simulink model "CompleteModel"  (R2015b)
settings: Solver=VariableStepAuto  StartTime=0.0  StopTime=t  RelTol=1e-3
undefined symbols (not defined in the file): Fg, Jx, Jy, Jz, kd, kth, L, m, w1_bar, w2_bar, w3_bar, w4_bar
libraries: simulink x6
settings Model: Creator=USUARIO  LastModifiedBy=USUARIO

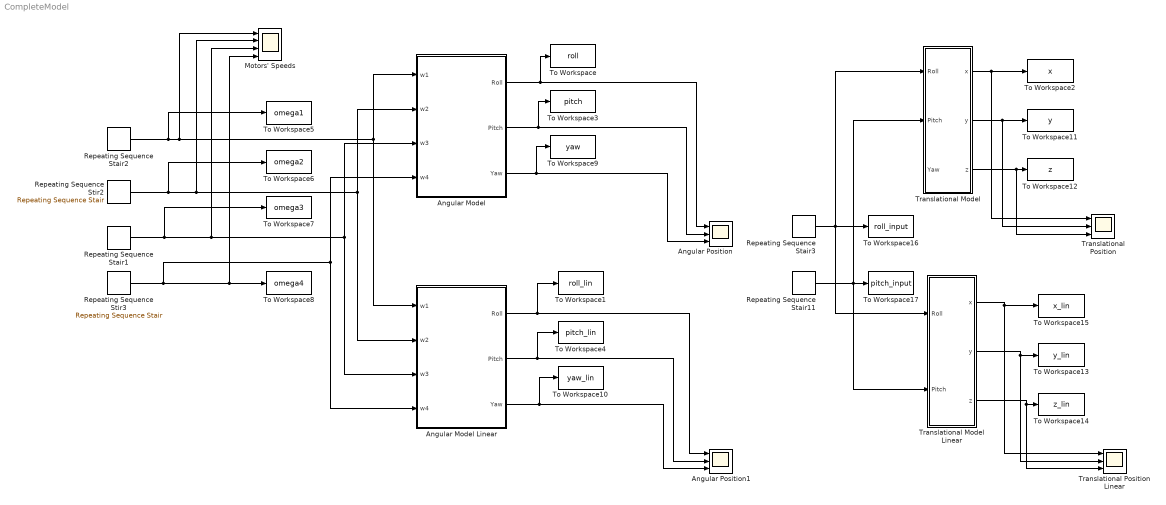
== system CompleteModel ==
  Angular Model : Subsystem
  Angular Model Linear : Subsystem
  Angular Position : Scope  NumInputPorts=3
  Angular Position1 : Scope  NumInputPorts=3
  Motors' Speeds : Scope  NumInputPorts=4
  Repeating Sequence Stair1 : simulink/Sources/Repeating Sequence Stair  OutValues=inputw3  tsamp=2  OutMin=[]  OutMax=[]  OutDataTypeStr=double  OutputDataTypeScalingMode=double  OutDataType=fixdt(0,8)  ConRadixGroup=Best Precision: Vector-wise  OutScaling=2^-12
  "Repeating Sequence Stair11 " : simulink/Sources/Repeating Sequence Stair  OutValues=inputpitch  tsamp=2  OutMin=[]  OutMax=[]  OutDataTypeStr=double  OutputDataTypeScalingMode=double  OutDataType=fixdt(0,8)  ConRadixGroup=Best Precision: Vector-wise  OutScaling=2^-12
  Repeating Sequence Stair2 : simulink/Sources/Repeating Sequence Stair  OutValues=inputw1  tsamp=2  OutMin=[]  OutMax=[]  OutDataTypeStr=double  OutputDataTypeScalingMode=double  OutDataType=fixdt(0,8)  ConRadixGroup=Best Precision: Vector-wise  OutScaling=2^-12
  Repeating Sequence Stair3 : simulink/Sources/Repeating Sequence Stair  OutValues=inputroll  tsamp=2  OutMin=[]  OutMax=[]  OutDataTypeStr=double  OutputDataTypeScalingMode=double  OutDataType=fixdt(0,8)  ConRadixGroup=Best Precision: Vector-wise  OutScaling=2^-12
  Repeating Sequence Stir2 : simulink/Sources/Repeating Sequence Stair  OutValues=inputw2  tsamp=2  OutMin=[]  OutMax=[]  OutDataTypeStr=double  OutputDataTypeScalingMode=double  OutDataType=fixdt(0,8)  ConRadixGroup=Best Precision: Vector-wise  OutScaling=2^-12
  Repeating Sequence Stir3 : simulink/Sources/Repeating Sequence Stair  OutValues=inputw4  tsamp=2  OutMin=[]  OutMax=[]  OutDataTypeStr=double  OutputDataTypeScalingMode=double  OutDataType=fixdt(0,8)  ConRadixGroup=Best Precision: Vector-wise  OutScaling=2^-12
  To Workspace : ToWorkspace  VariableName=roll  SaveFormat=Timeseries  SampleTime=0.1
  To Workspace1 : ToWorkspace  VariableName=roll_lin  SaveFormat=Timeseries  SampleTime=0.1
  To Workspace10 : ToWorkspace  VariableName=yaw_lin  SaveFormat=Timeseries  SampleTime=0.1
  To Workspace11 : ToWorkspace  VariableName=y  SaveFormat=Timeseries  SampleTime=0.1
  To Workspace12 : ToWorkspace  VariableName=z  SaveFormat=Timeseries  SampleTime=0.1
  To Workspace13 : ToWorkspace  VariableName=y_lin  SaveFormat=Timeseries  SampleTime=0.1
  To Workspace14 : ToWorkspace  VariableName=z_lin  SaveFormat=Timeseries  SampleTime=0.1
  To Workspace15 : ToWorkspace  VariableName=x_lin  SaveFormat=Timeseries  SampleTime=0.1
  To Workspace16 : ToWorkspace  VariableName=roll_input  SaveFormat=Timeseries  SampleTime=0.1
  To Workspace17 : ToWorkspace  VariableName=pitch_input  SaveFormat=Timeseries  SampleTime=0.1
  To Workspace2 : ToWorkspace  VariableName=x  SaveFormat=Timeseries  SampleTime=0.1
  To Workspace3 : ToWorkspace  VariableName=pitch  SaveFormat=Timeseries  SampleTime=0.1
  To Workspace4 : ToWorkspace  VariableName=pitch_lin  SaveFormat=Timeseries  SampleTime=0.1
  To Workspace5 : ToWorkspace  VariableName=omega1  SaveFormat=Timeseries  SampleTime=0.1
  To Workspace6 : ToWorkspace  VariableName=omega2  SaveFormat=Timeseries  SampleTime=0.1
  To Workspace7 : ToWorkspace  VariableName=omega3  SaveFormat=Timeseries  SampleTime=0.1
  To Workspace8 : ToWorkspace  VariableName=omega4  SaveFormat=Timeseries  SampleTime=0.1
  To Workspace9 : ToWorkspace  VariableName=yaw  SaveFormat=Timeseries  SampleTime=0.1
  Translational Model : Subsystem
  Translational Model Linear : Subsystem
  Translational Position : Scope  NumInputPorts=3
  Translational Position Linear : Scope  NumInputPorts=3
  wires:
  Angular Model/1(Roll) -> Angular Position/1, To Workspace/1
  Angular Model/2(Pitch) -> Angular Position/2, To Workspace3/1
  Angular Model/3(Yaw) -> To Workspace9/1, Angular Position/3
  Translational Model/1(x) -> To Workspace2/1, Translational Position/1
  Translational Model/2(y) -> To Workspace11/1, Translational Position/2
  Translational Model/3(z) -> Translational Position/3, To Workspace12/1
  Angular Model Linear/1(Roll) -> Angular Position1/1, To Workspace1/1
  Angular Model Linear/2(Pitch) -> To Workspace4/1, Angular Position1/2
  Angular Model Linear/3(Yaw) -> Angular Position1/3, To Workspace10/1
  Repeating Sequence Stir3/1 -> Motors' Speeds/4, To Workspace8/1, Angular Model/4(w4), Angular Model Linear/4(w4)
  Repeating Sequence Stair1/1 -> To Workspace7/1, Motors' Speeds/3, Angular Model/3(w3), Angular Model Linear/3(w3)
  Repeating Sequence Stir2/1 -> To Workspace6/1, Motors' Speeds/2, Angular Model Linear/2(w2), Angular Model/2(w2)
  Repeating Sequence Stair2/1 -> To Workspace5/1, Motors' Speeds/1, Angular Model Linear/1(w1), Angular Model/1(w1)
  Repeating Sequence Stair3/1 -> To Workspace16/1, Translational Model/1(Roll), Translational Model Linear/1(Roll)
  "Repeating Sequence Stair11 "/1 -> Translational Model/2(Pitch), To Workspace17/1, Translational Model Linear/2(Pitch)
  Translational Model Linear/1(x) -> Translational Position Linear/1, To Workspace15/1
  Translational Model Linear/2(y) -> Translational Position Linear/2, To Workspace13/1
  Translational Model Linear/3(z) -> Translational Position Linear/3, To Workspace14/1

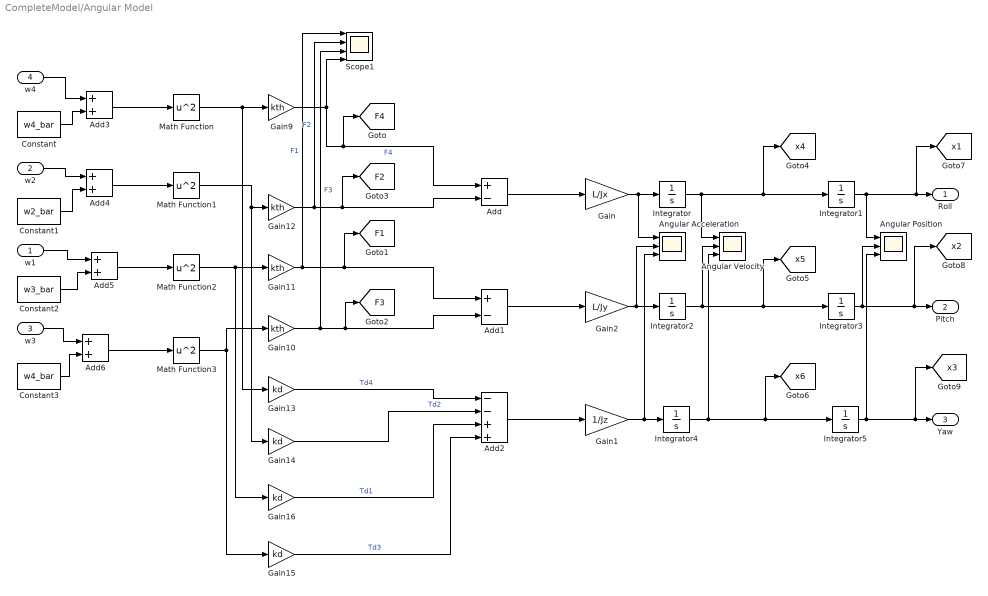
== system CompleteModel/Angular Model ==
  w1 : Inport
  w2 : Inport  Port=2
  w3 : Inport  Port=3
  w4 : Inport  Port=4
  Add : Sum  Inputs=+-
  Add1 : Sum  Inputs=+-
  Add2 : Sum  Inputs=--++
  Add{3..6} (4 alike) : Sum
  Angular Position : Scope  NumInputPorts=3
  Angular Velocity : Scope  NumInputPorts=3
  Angular Acceleration : Scope  NumInputPorts=3
  Constant : Constant  Value=w4_bar
  Constant1 : Constant  Value=w2_bar
  Constant2 : Constant  Value=w3_bar
  Constant3 : Constant  Value=w4_bar
  Gain : Gain  Gain=L/Jx
  Gain1 : Gain  Gain=1/Jz
  Gain{9..12} (4 alike) : Gain  Gain=kth
  Gain{13..16} (4 alike) : Gain  Gain=kd
  Gain2 : Gain  Gain=L/Jy
  Integrator{,1..5} (6 alike) : Integrator
  Math Function{,1..3} (4 alike) : Math  Operator=square  SaturateOnIntegerOverflow=on
  Scope1 : Scope  NumInputPorts=4
  Roll : Outport
  Pitch : Outport  Port=2
  Yaw : Outport  Port=3
  tag scope: F1=global, F2=global, F3=global, F4=global, x1=global, x2=global, x3=global, x4=global, x5=global, x6=global
  wires:
  Gain2/1 -> Angular Acceleration/2, Integrator2/1
  Add2/1 -> Gain1/1
  Gain9/1 -> [F4], Add/1, Scope1/4  "F4"
  Gain14/1 -> Add2/2  "Td2"
  Gain16/1 -> Add2/3  "Td1"
  Gain/1 -> Angular Acceleration/1, Integrator/1
  Integrator/1 -> Angular Velocity/1, Integrator1/1, [x4]
  Integrator1/1 -> [x1], Roll/1, Angular Position/1
  Integrator4/1 -> Angular Velocity/3, [x6], Integrator5/1
  Add/1 -> Gain/1
  Integrator3/1 -> [x2], Pitch/1, Angular Position/2
  Add1/1 -> Gain2/1
  Integrator5/1 -> Angular Position/3, [x3], Yaw/1
  Gain12/1 -> Scope1/2, [F2], Add/2  "F2"
  Gain10/1 -> [F3], Add1/2, Scope1/3  "F3"
  Gain11/1 -> Scope1/1, [F1], Add1/1  "F1"
  Gain13/1 -> Add2/1  "Td4"
  Gain15/1 -> Add2/4  "Td3"
  Integrator2/1 -> Angular Velocity/2, [x5], Integrator3/1
  Gain1/1 -> Angular Acceleration/3, Integrator4/1
  Math Function3/1 -> Gain10/1, Gain15/1
  Math Function2/1 -> Gain16/1, Gain11/1
  Math Function/1 -> Gain13/1, Gain9/1
  Math Function1/1 -> Gain14/1, Gain12/1
  w4/1 -> Add3/1
  Add3/1 -> Math Function/1
  Constant/1 -> Add3/2
  w2/1 -> Add4/1
  Add4/1 -> Math Function1/1
  Constant1/1 -> Add4/2
  w1/1 -> Add5/1
  Add5/1 -> Math Function2/1
  Constant2/1 -> Add5/2
  w3/1 -> Add6/1
  Add6/1 -> Math Function3/1
  Constant3/1 -> Add6/2

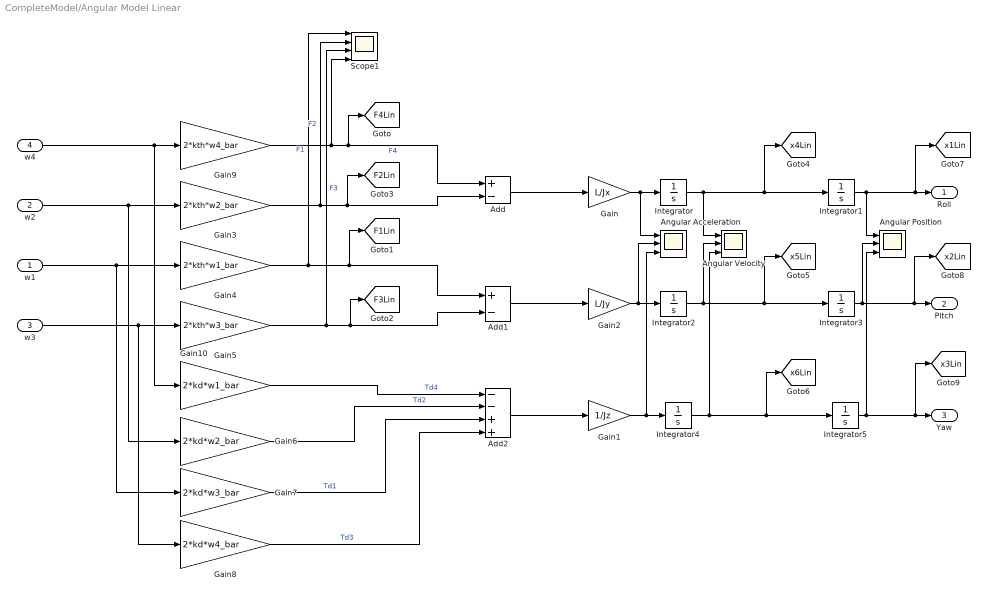
== system CompleteModel/Angular Model Linear ==
  w1 : Inport
  w2 : Inport  Port=2
  w3 : Inport  Port=3
  w4 : Inport  Port=4
  Add : Sum  Inputs=+-
  Add1 : Sum  Inputs=+-
  Add2 : Sum  Inputs=--++
  Angular Position : Scope  NumInputPorts=3
  Angular Velocity : Scope  NumInputPorts=3
  Angular Acceleration : Scope  NumInputPorts=3
  Gain : Gain  Gain=L/Jx
  Gain1 : Gain  Gain=1/Jz
  Gain10 : Gain  Gain=2*kd*w1_bar
  Gain2 : Gain  Gain=L/Jy
  Gain3 : Gain  Gain=2*kth*w2_bar
  Gain4 : Gain  Gain=2*kth*w1_bar
  Gain5 : Gain  Gain=2*kth*w3_bar
  Gain6 : Gain  Gain=2*kd*w2_bar
  Gain7 : Gain  Gain=2*kd*w3_bar
  Gain8 : Gain  Gain=2*kd*w4_bar
  Gain9 : Gain  Gain=2*kth*w4_bar
  Integrator{,1..5} (6 alike) : Integrator
  Scope1 : Scope  NumInputPorts=4
  Roll : Outport
  Pitch : Outport  Port=2
  Yaw : Outport  Port=3
  tag scope: F1Lin=global, F2Lin=global, F3Lin=global, F4Lin=global, x1Lin=global, x2Lin=global, x3Lin=global, x4Lin=global, x5Lin=global, x6Lin=global
  wires:
  w4/1 -> Gain10/1, Gain9/1
  w3/1 -> Gain5/1, Gain8/1
  Gain1/1 -> Integrator4/1, Angular Acceleration/3
  Integrator2/1 -> Integrator3/1, [x5Lin], Angular Velocity/2
  Gain8/1 -> Add2/4  "Td3"
  Gain10/1 -> Add2/1  "Td4"
  Gain4/1 -> Add1/1, [F1Lin], Scope1/1  "F1"
  Gain5/1 -> Scope1/3, Add1/2, [F3Lin]  "F3"
  Gain3/1 -> Scope1/2, Add/2, [F2Lin]  "F2"
  Integrator5/1 -> Yaw/1, [x3Lin], Angular Position/3
  Add1/1 -> Gain2/1
  Integrator3/1 -> Angular Position/2, Pitch/1, [x2Lin]
  Add/1 -> Gain/1
  Integrator4/1 -> Integrator5/1, [x6Lin], Angular Velocity/3
  Integrator1/1 -> Angular Position/1, Roll/1, [x1Lin]
  Integrator/1 -> [x4Lin], Integrator1/1, Angular Velocity/1
  Gain/1 -> Integrator/1, Angular Acceleration/1
  Gain7/1 -> Add2/3  "Td1"
  Gain6/1 -> Add2/2  "Td2"
  Gain9/1 -> Scope1/4, Add/1, [F4Lin]  "F4"
  Add2/1 -> Gain1/1
  Gain2/1 -> Integrator2/1, Angular Acceleration/2
  w2/1 -> Gain3/1, Gain6/1
  w1/1 -> Gain7/1, Gain4/1

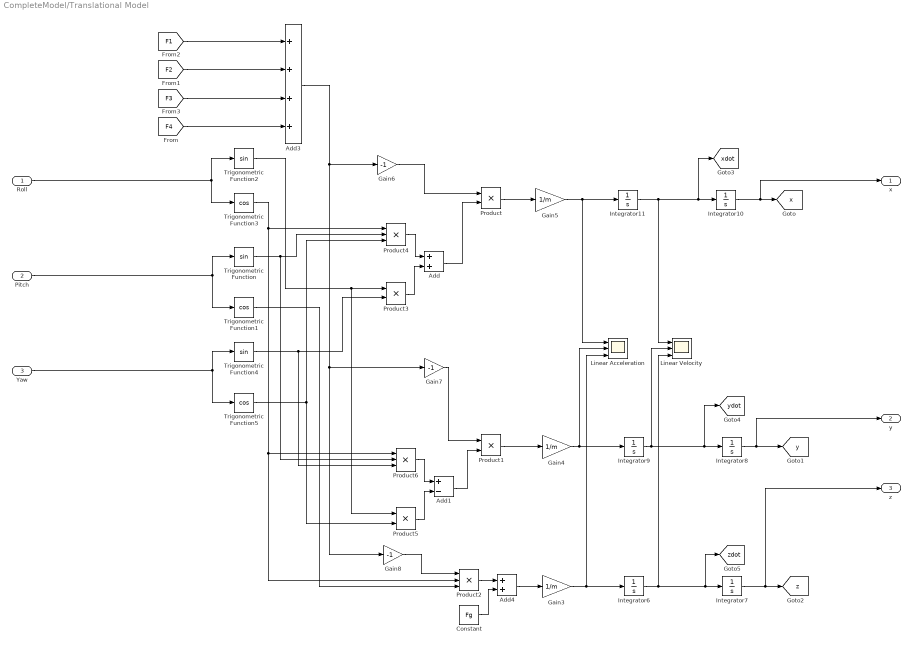
== system CompleteModel/Translational Model ==
  Roll : Inport
  Pitch : Inport  Port=2
  "Yaw " : Inport  Port=3
  Add : Sum
  Add1 : Sum  Inputs=+-
  Add3 : Sum  Inputs=4
  Add4 : Sum  Inputs=2
  Constant : Constant  Value=Fg
  Gain3 : Gain  Gain=1/m
  Gain4 : Gain  Gain=1/m
  Gain5 : Gain  Gain=1/m
  Gain6 : Gain  Gain=-1
  Gain7 : Gain  Gain=-1
  Gain8 : Gain  Gain=-1
  Integrator{6..11} (6 alike) : Integrator
  Linear Acceleration : Scope  NumInputPorts=3
  Linear Velocity : Scope  NumInputPorts=3
  Product{,1,3,5} (4 alike) : Product
  Product2 : Product  Inputs=3
  Product4 : Product  Inputs=3
  Product6 : Product  Inputs=3
  Trigonometric Function : Trigonometry
  Trigonometric Function1 : Trigonometry  Operator=cos
  Trigonometric Function2 : Trigonometry
  Trigonometric Function3 : Trigonometry  Operator=cos
  Trigonometric Function4 : Trigonometry
  Trigonometric Function5 : Trigonometry  Operator=cos
  x : Outport
  y : Outport  Port=2
  z : Outport  Port=3
  tag scope: x=global, xdot=global, y=global, ydot=global, z=global, zdot=global
  wires:
  Integrator11/1 -> [xdot], Integrator10/1, Linear Velocity/1
  Integrator7/1 -> z/1, [z]
  Gain5/1 -> Integrator11/1, Linear Acceleration/1
  Integrator9/1 -> [ydot], Integrator8/1, Linear Velocity/2
  Integrator10/1 -> [x], x/1
  Integrator8/1 -> y/1, [y]
  [F3] -> Add3/3
  Product/1 -> Gain5/1
  Product1/1 -> Gain4/1
  Gain4/1 -> Integrator9/1, Linear Acceleration/2
  Integrator6/1 -> [zdot], Integrator7/1, Linear Velocity/3
  Gain7/1 -> Product1/1
  Trigonometric Function2/1 -> Product5/1, Product3/1
  Constant/1 -> Add4/2
  [F4] -> Add3/4
  Add3/1 -> Gain8/1, Gain7/1, Gain6/1
  [F2] -> Add3/2
  Trigonometric Function1/1 -> Product2/3
  [F1] -> Add3/1
  Product2/1 -> Add4/1
  Add4/1 -> Gain3/1
  Gain6/1 -> Product/1
  Gain8/1 -> Product2/1
  Trigonometric Function3/1 -> Product4/1, Product6/1, Product2/2
  Gain3/1 -> Integrator6/1, Linear Acceleration/3
  Roll/1 -> Trigonometric Function3/1, Trigonometric Function2/1
  Pitch/1 -> Trigonometric Function/1, Trigonometric Function1/1
  Add/1 -> Product/2
  Product3/1 -> Add/2
  Product4/1 -> Add/1
  "Yaw "/1 -> Trigonometric Function4/1, Trigonometric Function5/1
  Trigonometric Function/1 -> Product6/2, Product4/2
  Trigonometric Function5/1 -> Product4/3, Product5/2
  Trigonometric Function4/1 -> Product6/3, Product3/2
  Product5/1 -> Add1/2
  Product6/1 -> Add1/1
  Add1/1 -> Product1/2

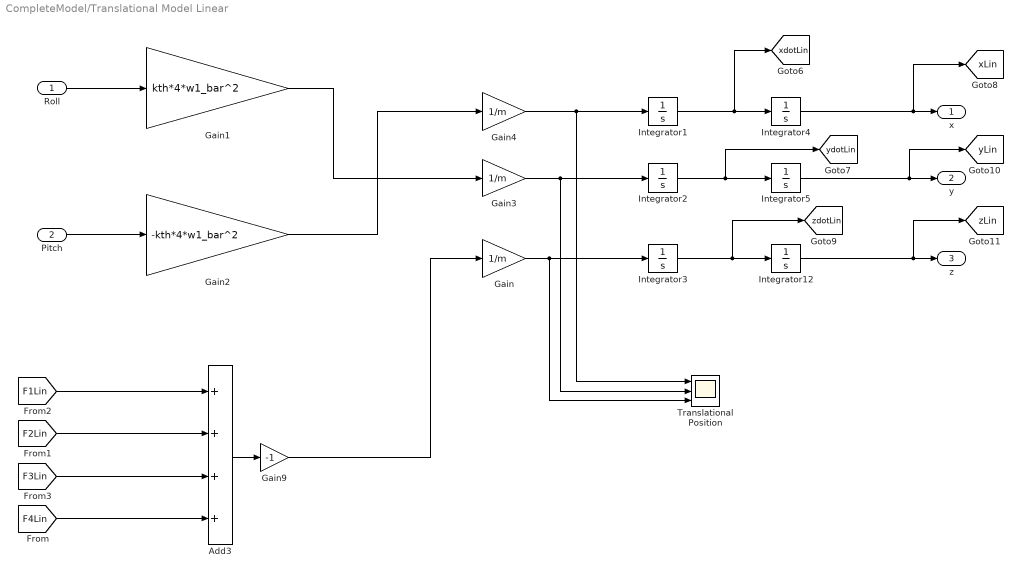
== system CompleteModel/Translational Model Linear ==
  Roll : Inport
  Pitch : Inport  Port=2
  Add3 : Sum  Inputs=4
  Gain : Gain  Gain=1/m
  Gain1 : Gain  Gain=kth*4*w1_bar^2
  Gain2 : Gain  Gain=-kth*4*w1_bar^2
  Gain3 : Gain  Gain=1/m
  Gain4 : Gain  Gain=1/m
  Gain9 : Gain  Gain=-1
  Integrator{1..5,12} (6 alike) : Integrator
  Translational Position : Scope  NumInputPorts=3
  x : Outport
  y : Outport  Port=2
  z : Outport  Port=3
  tag scope: xLin=global, xdotLin=global, yLin=global, ydotLin=global, zLin=global, zdotLin=global
  wires:
  [F1Lin] -> Add3/1
  [F2Lin] -> Add3/2
  [F4Lin] -> Add3/4
  [F3Lin] -> Add3/3
  Add3/1 -> Gain9/1
  Gain2/1 -> Gain4/1
  Gain1/1 -> Gain3/1
  Roll/1 -> Gain1/1
  Pitch/1 -> Gain2/1
  Integrator1/1 -> [xdotLin], Integrator4/1
  Integrator2/1 -> [ydotLin], Integrator5/1
  Integrator3/1 -> [zdotLin], Integrator12/1
  Integrator4/1 -> [xLin], x/1
  Integrator5/1 -> [yLin], y/1
  Integrator12/1 -> [zLin], z/1
  Gain9/1 -> Gain/1
  Gain/1 -> Integrator3/1, Translational Position/3
  Gain3/1 -> Integrator2/1, Translational Position/2
  Gain4/1 -> Integrator1/1, Translational Position/1
